simulink model "CA4_Q1_lastPart"  (R2020a)
settings: Solver=VariableStepAuto  StartTime=0.0  StopTime=10.0  RelTol=1e-3
settings Model: Creator=golnazsalehi  LastModifiedBy=golnazsalehi

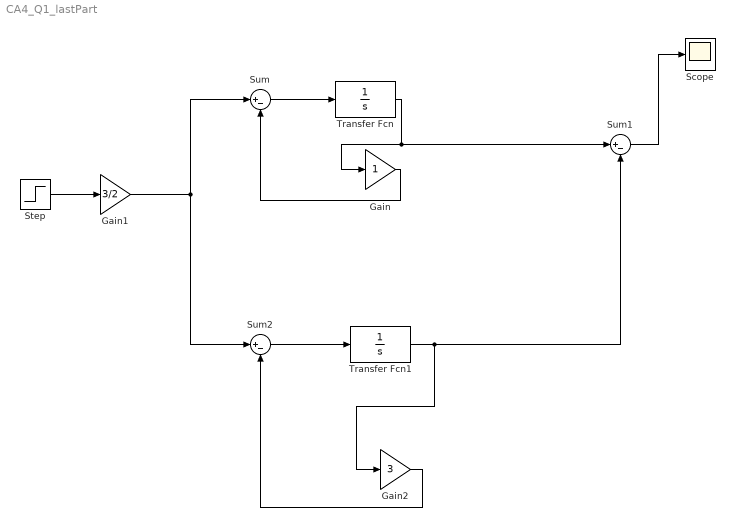
== system CA4_Q1_lastPart ==
  Gain : Gain
  Gain1 : Gain  Gain=3/2
  Gain2 : Gain  Gain=3
  Scope : Scope
  Step : Step  Time=0  SampleTime=0
  Sum : Sum  Inputs=|+-
  Sum1 : Sum  Inputs=|+-
  Sum2 : Sum  Inputs=|+-
  Transfer Fcn : TransferFcn  Denominator=[1 0]
  Transfer Fcn1 : TransferFcn  Denominator=[1 0]
  wires:
  Transfer Fcn/1 -> Sum1/1, Gain/1
  Gain/1 -> Sum/2
  Sum/1 -> Transfer Fcn/1
  Step/1 -> Gain1/1
  Gain1/1 -> Sum2/1, Sum/1
  Transfer Fcn1/1 -> Sum1/2, Gain2/1
  Gain2/1 -> Sum2/2
  Sum2/1 -> Transfer Fcn1/1
  Sum1/1 -> Scope/1
